simulink library "vmc"  (R2021b)
settings: Solver=VariableStepAuto  StartTime=0.0  StopTime=10.0  RelTol=1e-3
undefined symbols (not defined in the file): AVMC_ACCDeltaTqGradeGn_X_deg, AVMC_ACCDeltaTqIGain4OVRD_X_kph, AVMC_ACCDeltaTqIGain4OVRD_Y_mps2, AVMC_ACCDeltaTqIGain_X_kph, AVMC_ACCDeltaTqIGain_Y_mps2, AVMC_ACCDeltaTqPGain_X_kph, AVMC_ACCDeltaTqPGain_Y_kph, AVMC_ACCGradeofst_X_G, AVMC_ACCGradeofst_Y_pct, AVMC_ACCLoSpdTqLoLim4JP_X_kph, AVMC_ACCLoSpdTqLoLim4JP_Y_deg, AVMC_ACCLoSpdTqLowerLim_X_kph, AVMC_ACCLoSpdTqLowerLim_Y_deg, AVMC_ACCReqAccelGain_X_mps2, AVMC_ACCReqAccelGain_Y_enum, AVMC_ADSPosGFBDeltaTq_X_kph, AVMC_ADSPosGFBDeltaTq_Y_mps2, AVMC_AggressJerkPCT4AT_X_kph, AVMC_AggressJerkPCT_X_kph, AVMC_AggressLimitPCT4AT_X_kph, AVMC_AggressLimitPCT_X_kph, AVMC_DECGradeofst_X_G, AVMC_DECGradeofst_Y_pct, AVMC_DISCDeltaTqIGain_X_kph, AVMC_DISCDeltaTqIGain_Y_mps2, AVMC_DISCDeltaTqPGain_X_kph, AVMC_DISCDeltaTqPGain_Y_kph, AVMC_EPSForceSelect_X_enum, AVMC_EPSForceSelect_Y_enum, AVMC_EPSForceSelectD21_X_enum, AVMC_EPSForceSelectD21_Y_enum, AVMC_ESCRegenOut_X_kph, AVMC_ESCRegenOut_Y_Deg, AVMC_ESCRegenOutEnSpd_X_Deg, AVMC_EstPitchSlopeTs_X_kph, AVMC_GradeCompFlt_X_kph, AVMC_GyroYBandLo_X_Gps, AVMC_HoldResTq_X_kph, AVMC_ISOAccLimit_X_mps, AVMC_ISODecLimit_X_mps, AVMC_ISOJerk_X_mps, AVMC_LatESCRegenOut_X_kph, AVMC_LatESCRegenOut_Y_Deg, AVMC_LongAccDeadZone_X_kph, AVMC_LongAccFiltTsforP2_X_Gps, AVMC_MCPresBaseTq_X_bar, AVMC_MSAPedalOvrd_X_kph, AVMC_MSASpdBand_X_kph, AVMC_MSATqDownEndTq_X_kph, AVMC_MSATqDownTime_X_kph, AVMC_NegZCHoldTq_X_kph, AVMC_OPDDisSlideRate_X_Deg, AVMC_OVRD2ActSR2FCMCMD_X_mps2, AVMC_PedalTqRWhlRatio_X_Nm, AVMC_PedalTqRWhlRatio_Y_gps, AVMC_PedalTqRWhlSlipGain_X_rat, AVMC_PedalTqRWhlSlipGain_Y_kph, AVMC_PedalTqRWhSTRGGain_X_deg, AVMC_PedalTqRWhSTRGGain_Y_kph, AVMC_PosZCHoldTq_X_kph ... (+593)
libraries: hcu_lib x143, simulink x96, tqr x4, $bdroot x1, simulink_extras x1
(part 13 of 17)

== system vmc/VMC/VMC/SPD2ACC/SPD2ACC Active Determination ==
  VVMC_FeatArbitrSta_enum : Inport
  Constant : Constant  Value=TRUE
  Constant1 : Constant  Value=FALSE
  Constant13 : Constant  Value=ENUM_FEATARBITRSTA_DISC
  Constant2 : Constant  Value=ENUM_FEATARBITRSTA_ACCDISC
  Constant3 : Constant  Value=ENUM_FEATARBITRSTA_CC
  Constant4 : Constant  Value=ENUM_FEATARBITRSTA_MSA
  SPD2ACC Active Determination : Stateflow chart  TreatAsAtomicUnit=on
  VVMC_SPD2ACCAct_flg : Outport
  wires:
  Constant4/1 -> SPD2ACC Active Determination/7(ENUM_FEATARBITRSTA_MSA)
  Constant3/1 -> SPD2ACC Active Determination/6(ENUM_FEATARBITRSTA_CC)
  VVMC_FeatArbitrSta_enum/1 -> [VVMC_FeatArbitrSta_enum]
  [VVMC_FeatArbitrSta_enum] -> SPD2ACC Active Determination/1(VVMC_FeatArbitrSta_enum)
  SPD2ACC Active Determination/1(VVMC_SPD2ACCAct_flg) -> [VVMC_SPD2ACCAct_flg]
  [VVMC_SPD2ACCAct_flg] -> VVMC_SPD2ACCAct_flg/1
  Constant/1 -> SPD2ACC Active Determination/2(TURE)
  Constant1/1 -> SPD2ACC Active Determination/3(FALSE)
  Constant13/1 -> SPD2ACC Active Determination/4(ENUM_FEATARBITRSTA_DISC)
  Constant2/1 -> SPD2ACC Active Determination/5(ENUM_FEATARBITRSTA_ACCDISC)

== system vmc/VMC/VMC/SafetyControl/ADB_VehPitchAngleSta ==
  VVMC_CalibratedAccXAftRA_G : Inport
  task_time_s : Inport  Port=2
  VTQD_ExtDoorAllow_flg : Inport  Port=3
  VVMC_VehicleSpeed_kph : Inport  Port=4
  VINP_GRADE_deg : Inport  Port=5
  2-D Lookup Table : Lookup_n-D  BreakpointsForDimension1=AVMC_VehPitchAngleSta_Y_deg  BreakpointsForDimension2=AVMC_VehPitchAngleSta_X_deg  Table=MVMC_VehPitchAngleSta_Z_enum  TableDataTypeStr=uint8  InterpMethod=Flat  InternalRulePriority=Speed  RndMeth=Simplest  InputSameDT=on
      settings: InputPortMap=u0,u1
  AND1 : Logic  AllPortsSameDT=off  OutDataTypeStr=boolean
  Asin : Trigonometry  Operator=asin
  Cast To Single6 : DataTypeConversion  OutDataTypeStr=uint8
  Constant14 : Constant  Value=KVMC_VehStandstillTimer_s
  Constant20 : Constant  Value=KVMC_VehStandstillSpd_kph
  Constant21 : Constant  Value=KVMC_VehPitchAngleMin_deg
  Constant27 : Constant  Value=KVMC_VehPitchAngleMax_deg
  Constant28 : Constant  Value=MINUSONE_FLOAT
  Constant29 : Constant  Value=ONE_FLOAT
  Constant3 : Constant  Value=KVMC_IMUGxFilter4ADB_raw32
  Constant4 : Constant  Value=KVMC_CalEstPitchAngleTs_raw32
  DelayEnable : hcu_lib/Basic_Blocks/DelayEnable
  Detect Increase1 : simulink/Logic and Bit Operations/Detect Increase  vinit=0.0  OutDataTypeStr=boolean
  FirstOrderFilter5 : hcu_lib/Basic_Blocks/FirstOrderFilter
  FirstOrderFilter7 : hcu_lib/Basic_Blocks/FirstOrderFilter
  Gain2 : Gain  Gain=RAD2DEG
  NOT : Logic  Operator=NOT  AllPortsSameDT=off  OutDataTypeStr=boolean
  Relational Operator1 : RelationalOperator  Operator=<  OutDataTypeStr=boolean  RndMeth=Simplest
  Relational Operator2 : RelationalOperator  Operator=<=  OutDataTypeStr=boolean  RndMeth=Simplest
  Relational Operator3 : RelationalOperator  OutDataTypeStr=boolean  RndMeth=Simplest
  SR_Latch4 : hcu_lib/Basic_Blocks/SR_Latch
  Saturation Dynamic3 : simulink/Discontinuities/Saturation Dynamic  OutMin=[]  OutMax=[]  OutDataTypeStr=Inherit: Same as second input  OutDataType=fixdt(1, 16)  OutScaling=2^-10  DoSatur=off
  Switch4 : Switch  Criteria=u2 > Threshold
  Switch5 : Switch  Criteria=u2 > Threshold
  Switch6 : Switch  Criteria=u2 > Threshold
  Unit Delay : UnitDelay  SampleTime=-1  HasFrameUpgradeWarning=on
  VVMC_VehPitchAngleSta_enum : Outport
  wires:
  [VVMC_MemVehPitchAngleEst_deg] -> Switch5/1
  Constant21/1 -> Relational Operator2/2
  Constant14/1 -> DelayEnable/2
  AND1/1 -> NOT/1, SR_Latch4/1
  Unit Delay/1 -> [VVMC_MemVehPitchAngleEst_deg]  "VVMC_MemVehPitchAngleEst_deg"
  Constant4/1 -> FirstOrderFilter7/3
  Constant20/1 -> Relational Operator1/2
  Constant3/1 -> FirstOrderFilter5/3
  FirstOrderFilter7/1 -> Switch4/1  "VVMC_CalEstPitchAngle_deg"
  DelayEnable/1 -> Detect Increase1/1
  Gain2/1 -> FirstOrderFilter7/1
  Asin/1 -> Gain2/1
  Relational Operator3/1 -> Switch6/2
  Switch5/1 -> Switch6/3, Relational Operator3/1
  [VVMC_VehPitchAngleEst_deg] -> 2-D Lookup Table/2
  SR_Latch4/1 -> DelayEnable/1  "VVMC_VehPitchAngleUpdCond_flg"
  [VVMC_VehicleSpeed_kph] -> Relational Operator1/1
  2-D Lookup Table/1 -> Cast To Single6/1
  [VVMC_MemVehPitchAngleEst_deg] -> Switch6/1
  Relational Operator2/1 -> Switch5/2
  Switch4/1 -> Switch5/3, Relational Operator2/1
  Cast To Single6/1 -> [VVMC_VehPitchAngleSta_enum]  "VVMC_VehPitchAngleSta_enum"
  Relational Operator1/1 -> AND1/2
  Switch6/1 -> Unit Delay/1, [VVMC_VehPitchAngleEst_deg]  "VVMC_VehPitchAngleEst_deg"
  [task_time_s] -> FirstOrderFilter7/2
  Detect Increase1/1 -> Switch4/2  "VVMC_VehPitchAngleUpd_flg"
  [VTQD_ExtDoorAllow_flg] -> AND1/1
  [task_time_s] -> DelayEnable/3
  [VVMC_MemVehPitchAngleEst_deg] -> Switch4/3
  [VVMC_CalibratedAccXAftRA_G] -> FirstOrderFilter5/1
  [VINP_GRADE_deg] -> 2-D Lookup Table/1
  [task_time_s] -> FirstOrderFilter5/2
  NOT/1 -> SR_Latch4/2
  Constant27/1 -> Relational Operator3/2
  [VVMC_VehPitchAngleSta_enum] -> VVMC_VehPitchAngleSta_enum/1
  VVMC_CalibratedAccXAftRA_G/1 -> [VVMC_CalibratedAccXAftRA_G]
  task_time_s/1 -> [task_time_s]
  VTQD_ExtDoorAllow_flg/1 -> [VTQD_ExtDoorAllow_flg]
  VVMC_VehicleSpeed_kph/1 -> [VVMC_VehicleSpeed_kph]
  VINP_GRADE_deg/1 -> [VINP_GRADE_deg]
  Constant29/1 -> Saturation Dynamic3/1
  Constant28/1 -> Saturation Dynamic3/3
  FirstOrderFilter5/1 -> Saturation Dynamic3/2
  Saturation Dynamic3/1 -> Asin/1

== system vmc/VMC/VMC/SafetyControl/LatAccRollingAverage ==
  VINP_LatAccel_Gps : Inport
  VINP_LatAccelV_flg : Inport  Port=2
  VDDM_ESC5Err_flg : Inport  Port=3
  Cast To Single4 : DataTypeConversion  OutDataTypeStr=uint8
  Constant15 : Constant  Value=ZERO_FLOAT
  Constant3 : Constant  Value=ONE_INT
  Constant4 : Constant  Value=ZERO_FLOAT
  Constant5 : Constant  Value=KVMC_LatAccRollAveLevel_enum
  Constant6 : Constant  Value=ONE_INT
  Min2 : MinMax  Function=max  Inputs=2
  OR2 : Logic  Operator=OR  AllPortsSameDT=off  OutDataTypeStr=boolean
  RollingAverage : Stateflow chart  TreatAsAtomicUnit=on
  Switch2 : Switch  Criteria=u2 > Threshold
  VVMC_LatAccRollAveRaw_Gps : Outport
  wires:
  [VDDM_ESC5Err_flg] -> OR2/2
  OR2/1 -> Switch2/2
  VDDM_ESC5Err_flg/1 -> [VDDM_ESC5Err_flg]
  [VINP_LatAccel_Gps] -> Switch2/3
  Constant15/1 -> Switch2/1
  [VINP_LatAccelV_flg] -> OR2/1
  VINP_LatAccelV_flg/1 -> [VINP_LatAccelV_flg]
  Cast To Single4/1 -> Min2/1
  Constant5/1 -> Cast To Single4/1
  Constant6/1 -> Min2/2
  Switch2/1 -> RollingAverage/4(VINP_LatAccel_Gps)
  Constant4/1 -> RollingAverage/2(ZERO_FLOAT)
  Constant3/1 -> RollingAverage/3(ONE_INT)
  Min2/1 -> RollingAverage/1(KVMC_LatAccRollAveLevel_enum)
  [VVMC_LatAccRollAveRaw_Gps] -> VVMC_LatAccRollAveRaw_Gps/1
  VINP_LatAccel_Gps/1 -> [VINP_LatAccel_Gps]
  RollingAverage/1(VVMC_LatAccRollAveRaw_Gps) -> [VVMC_LatAccRollAveRaw_Gps]  "VVMC_LatAccRollAveRaw_Gps"

== system vmc/VMC/VMC/SafetyControl/LongAccel_EstSlope_FrontRearSlipSpd ==
  VVMC_VehSpdRollAve_kph : Inport
  VVMC_CalibratedAccX_G : Inport  Port=2
  VVMC_IMUEnaCmd_flg : Inport  Port=3
  VINP_LongAccel_Gps : Inport  Port=4
  VINP_GRADE_deg : Inport  Port=5
  VVMC_LFWhlSpeedRollAve_kph : Inport  Port=6
  VVMC_RFWhlSpeedRollAve_kph : Inport  Port=7
  VVMC_LRWhlSpeedRollAve_kph : Inport  Port=8
  VVMC_RRWhlSpeedRollAve_kph : Inport  Port=9
  VINP_LFRawWhlSpeedV_flg : Inport  Port=10
  VINP_RFRawWhlSpeedV_flg : Inport  Port=11
  VINP_LRRawWhlSpeedV_flg : Inport  Port=12
  VINP_RRRawWhlSpeedV_flg : Inport  Port=13
  VVMC_VehicleSpeed_kph : Inport  Port=14
  task_time_s : Inport  Port=15
  AND : Logic  AllPortsSameDT=off  OutDataTypeStr=boolean
  Add1 : Sum
  Add10 : Sum  Inputs=+-
  Add9 : Sum
  Constant : Constant  Tag=struct('comment',struct('text','','placement',1),'output',struct('width',1,'name','$S_$B','unit','','type','Int16','offset',0,'max',NaN,'min',NaN,'freeze',1,'lsb',1,'arb',0,'class','default','address','','description','','value','0','tolerance',1,'show',0),'date',731450.689904282)  Value=ZERO_FLOAT  OutDataTypeStr=single
  Constant1 : Constant  Value=KVMC_LongAccelDiffTime_s
  Constant10 : Constant  Value=KVMC_LongAccelDiffTime_s
  Constant11 : Constant  Value=GRAVITY_G
  Constant12 : Constant  Value=KPH2MPS
  Constant13 : Constant  Tag=struct('comment',struct('text','','placement',1),'output',struct('width',1,'name','$S_$B','unit','','type','Int16','offset',0,'max',NaN,'min',NaN,'freeze',1,'lsb',1,'arb',0,'class','default','address','','description','','value','2','tolerance',1,'show',0),'date',731450.690075)  Value=TRUE
  Constant18 : Constant  Value=TWO_FLOAT
  Constant19 : Constant  Value=TWO_FLOAT
  Constant2 : Constant  Value=ZERO_FLOAT
  Constant24 : Constant  Value=GRAVITY_G
  Constant25 : Constant  Value=KPH2MPS
  Constant28 : Constant  Value=KVMC_EstSlopeGxSource_flg
  Constant3 : Constant  Tag=struct('comment',struct('text','','placement',1),'output',struct('width',1,'name','$S_$B','unit','','type','Int16','offset',0,'max',NaN,'min',NaN,'freeze',1,'lsb',1,'arb',0,'class','default','address','','description','','value','0','tolerance',1,'show',0),'date',731450.689904282)  Value=ZERO_FLOAT  OutDataTypeStr=single
  Constant4 : Constant  Value=KVMC_LongAccelDiffTime_s
  Constant5 : Constant  Tag=struct('comment',struct('text','','placement',1),'output',struct('width',1,'name','$S_$B','unit','','type','Int16','offset',0,'max',NaN,'min',NaN,'freeze',1,'lsb',1,'arb',0,'class','default','address','','description','','value','2','tolerance',1,'show',0),'date',731450.690075)  Value=TRUE
  Constant6 : Constant  Value=GRAVITY_G
  Constant7 : Constant  Value=KPH2MPS
  Constant8 : Constant  Tag=struct('comment',struct('text','','placement',1),'output',struct('width',1,'name','$S_$B','unit','','type','Int16','offset',0,'max',NaN,'min',NaN,'freeze',1,'lsb',1,'arb',0,'class','default','address','','description','','value','2','tolerance',1,'show',0),'date',731450.690075)  Value=TRUE
  Constant9 : Constant  Tag=struct('comment',struct('text','','placement',1),'output',struct('width',1,'name','$S_$B','unit','','type','Int16','offset',0,'max',NaN,'min',NaN,'freeze',1,'lsb',1,'arb',0,'class','default','address','','description','','value','0','tolerance',1,'show',0),'date',731450.689904282)  Value=ZERO_FLOAT  OutDataTypeStr=single
  Divide1 : Product  Inputs=**
  Divide2 : Product  Inputs=**
  Divide{3..6,8} (5 alike) : Product  Inputs=*/
  Divide7 : Product  Inputs=**
  Estimate Slope : Subsystem
  Max : MinMax  Function=max  Inputs=2
  Max1 : MinMax  Function=max  Inputs=2
  Max2 : MinMax  Function=max  Inputs=2
  OR1 : Logic  Operator=OR  AllPortsSameDT=off  OutDataTypeStr=boolean
  OR2 : Logic  Operator=OR  AllPortsSameDT=off  OutDataTypeStr=boolean
  OR3 : Logic  AllPortsSameDT=off  OutDataTypeStr=boolean
  OR4 : Logic  AllPortsSameDT=off  OutDataTypeStr=boolean
  OR5 : Logic  Operator=OR  AllPortsSameDT=off  OutDataTypeStr=boolean
  Product : Product  Tag=struct('comment',struct('text','','placement',1),'logdata',struct('maxnumvals',inf,'plotchannels',[],'stepsize',0,'downsampling',1,'loggingmode',3,'channels',1),'output',struct('width',1,'name','$S_$B','unit','','type','Int32Bin15','offset',0,'max',65535,'min',-65536,'freeze',1,'lsb',2^-15,'arb',0,'class','default','address','','description','','autoscalingmode',1,'lowerheadroom',1,'upperheadroom',1,'headroomunit','bit','checkmin',0,'checkmax',0,'show',0),'inputs','*/','exceptionhandling',1,'date',731458.438505301)  Inputs=*/  InputSameDT=on  RndMeth=Zero  SaturateOnIntegerOverflow=on  OutDataTypeStr=Inherit: Same as first input
  Product1 : Product  Tag=struct('comment',struct('text','','placement',1),'logdata',struct('maxnumvals',inf,'plotchannels',[],'stepsize',0,'downsampling',1,'loggingmode',3,'channels',1),'output',struct('width',1,'name','$S_$B','unit','','type','Int32Bin15','offset',0,'max',65535,'min',-65536,'freeze',1,'lsb',2^-15,'arb',0,'class','default','address','','description','','autoscalingmode',1,'lowerheadroom',1,'upperheadroom',1,'headroomunit','bit','checkmin',0,'checkmax',0,'show',0),'inputs','*/','exceptionhandling',1,'date',731458.438505301)  Inputs=*/  InputSameDT=on  RndMeth=Zero  SaturateOnIntegerOverflow=on  OutDataTypeStr=Inherit: Same as first input
  Product2 : Product  Tag=struct('comment',struct('text','','placement',1),'logdata',struct('maxnumvals',inf,'plotchannels',[],'stepsize',0,'downsampling',1,'loggingmode',3,'channels',1),'output',struct('width',1,'name','$S_$B','unit','','type','Int32Bin15','offset',0,'max',65535,'min',-65536,'freeze',1,'lsb',2^-15,'arb',0,'class','default','address','','description','','autoscalingmode',1,'lowerheadroom',1,'upperheadroom',1,'headroomunit','bit','checkmin',0,'checkmax',0,'show',0),'inputs','*/','exceptionhandling',1,'date',731458.438505301)  Inputs=*/  InputSameDT=on  RndMeth=Zero  SaturateOnIntegerOverflow=on  OutDataTypeStr=Inherit: Same as first input
  Sum : Sum  Tag=struct('comment',struct('text','','placement',1),'logdata',struct('maxnumvals',inf,'plotchannels',[],'stepsize',0,'downsampling',1,'loggingmode',3,'channels',1),'output',struct('width',1,'name','$S_$B','unit','','type','Int32Bin15','offset',0,'max',65535,'min',-65536,'freeze',1,'lsb',2^-15,'arb',0,'class','default','address','','description','','autoscalingmode',1,'lowerheadroom',1,'upperheadroom',1,'headroomunit','bit','checkmin',0,'checkmax',0,'show',0),'inputs','+-','date',731450.688943275)  Inputs=+-  InputSameDT=on  SaturateOnIntegerOverflow=on  OutDataTypeStr=Inherit: Same as first input
  Sum1 : Sum  Tag=struct('comment',struct('text','','placement',1),'logdata',struct('maxnumvals',inf,'plotchannels',[],'stepsize',0,'downsampling',1,'loggingmode',3,'channels',1),'output',struct('width',1,'name','$S_$B','unit','','type','Int32Bin15','offset',0,'max',65535,'min',-65536,'freeze',1,'lsb',2^-15,'arb',0,'class','default','address','','description','','autoscalingmode',1,'lowerheadroom',1,'upperheadroom',1,'headroomunit','bit','checkmin',0,'checkmax',0,'show',0),'inputs','+-','date',731450.688943275)  Inputs=+-  InputSameDT=on  SaturateOnIntegerOverflow=on  OutDataTypeStr=Inherit: Same as first input
  Sum2 : Sum  Tag=struct('comment',struct('text','','placement',1),'logdata',struct('maxnumvals',inf,'plotchannels',[],'stepsize',0,'downsampling',1,'loggingmode',3,'channels',1),'output',struct('width',1,'name','$S_$B','unit','','type','Int32Bin15','offset',0,'max',65535,'min',-65536,'freeze',1,'lsb',2^-15,'arb',0,'class','default','address','','description','','autoscalingmode',1,'lowerheadroom',1,'upperheadroom',1,'headroomunit','bit','checkmin',0,'checkmax',0,'show',0),'inputs','+-','date',731450.688943275)  Inputs=+-  InputSameDT=on  SaturateOnIntegerOverflow=on  OutDataTypeStr=Inherit: Same as first input
  Switch{,1..3} (4 alike) : Switch  Criteria=u2 > Threshold
  Switch4 : Switch  Tag=struct('comment',struct('text','','placement',1),'logdata',struct('maxnumvals',inf,'plotchannels',[],'stepsize',0,'downsampling',1,'loggingmode',3,'channels',1),'output',struct('width',1,'name','$S_$B','unit','','type','Int32Bin15','offset',0,'max',65535,'min',-65536,'freeze',1,'lsb',2^-15,'arb',0,'class','default','address','','description','','autoscalingmode',1,'lowerheadroom',1,'upperheadroom',1,'headroomunit','bit','checkmin',0,'checkmax',0,'show',0),'threshold',struct('width',1,'name','$S_$B_threshold','unit','','type','Int16','offset',0,'max',NaN,'min',NaN,'freeze',1,'lsb',1,'arb',0,'class','default','address','','description','','value','1','scalar',0),'date',731458.438569977)  Criteria=u2 > Threshold  SaturateOnIntegerOverflow=on  InputSameDT=on
  Switch5 : Switch  Tag=struct('comment',struct('text','','placement',1),'logdata',struct('maxnumvals',inf,'plotchannels',[],'stepsize',0,'downsampling',1,'loggingmode',3,'channels',1),'output',struct('width',1,'name','$S_$B','unit','','type','Int32Bin15','offset',0,'max',65535,'min',-65536,'freeze',1,'lsb',2^-15,'arb',0,'class','default','address','','description','','autoscalingmode',1,'lowerheadroom',1,'upperheadroom',1,'headroomunit','bit','checkmin',0,'checkmax',0,'show',0),'threshold',struct('width',1,'name','$S_$B_threshold','unit','','type','Int16','offset',0,'max',NaN,'min',NaN,'freeze',1,'lsb',1,'arb',0,'class','default','address','','description','','value','1','scalar',0),'date',731458.438569977)  Criteria=u2 > Threshold  SaturateOnIntegerOverflow=on  InputSameDT=on
  Switch6 : Switch  Tag=struct('comment',struct('text','','placement',1),'logdata',struct('maxnumvals',inf,'plotchannels',[],'stepsize',0,'downsampling',1,'loggingmode',3,'channels',1),'output',struct('width',1,'name','$S_$B','unit','','type','Int32Bin15','offset',0,'max',65535,'min',-65536,'freeze',1,'lsb',2^-15,'arb',0,'class','default','address','','description','','autoscalingmode',1,'lowerheadroom',1,'upperheadroom',1,'headroomunit','bit','checkmin',0,'checkmax',0,'show',0),'threshold',struct('width',1,'name','$S_$B_threshold','unit','','type','Int16','offset',0,'max',NaN,'min',NaN,'freeze',1,'lsb',1,'arb',0,'class','default','address','','description','','value','1','scalar',0),'date',731458.438569977)  Criteria=u2 > Threshold  SaturateOnIntegerOverflow=on  InputSameDT=on
  UnitDelay1 : UnitDelay  Tag=struct('comment',struct('text','','placement',1),'logdata',struct('maxnumvals',inf,'plotchannels',[],'stepsize',0,'downsampling',1,'loggingmode',3,'channels',1),'output',struct('width',1,'name','$S_$B','unit','','type','Int32Bin15','offset',0,'max',65535,'min',-65536,'freeze',1,'lsb',2^-15,'arb',0,'class','default','address','','description','','autoscalingmode',1,'lowerheadroom',1,'upperheadroom',1,'headroomunit','bit','checkmin',0,'checkmax',0,'show',0,'initial','0'),'state',0,'dt','-1','date',731450.687911019)  SampleTime=-1  HasFrameUpgradeWarning=on
  UnitDelay2 : UnitDelay  Tag=struct('comment',struct('text','','placement',1),'logdata',struct('maxnumvals',inf,'plotchannels',[],'stepsize',0,'downsampling',1,'loggingmode',3,'channels',1),'output',struct('width',1,'name','$S_$B','unit','','type','UInt8','offset',0,'max',255,'min',0,'freeze',1,'lsb',1,'arb',0,'class','default','address','','description','','autoscalingmode',1,'lowerheadroom',1,'upperheadroom',1,'headroomunit','bit','checkmin',0,'checkmax',0,'show',0,'initial','0'),'state',0,'dt','-1','date',731450.690382801)  InitialCondition=FALSE  SampleTime=-1  StateName=first_pass  HasFrameUpgradeWarning=on
  UnitDelay3 : UnitDelay  Tag=struct('comment',struct('text','','placement',1),'logdata',struct('maxnumvals',inf,'plotchannels',[],'stepsize',0,'downsampling',1,'loggingmode',3,'channels',1),'output',struct('width',1,'name','$S_$B','unit','','type','Int32Bin15','offset',0,'max',65535,'min',-65536,'freeze',1,'lsb',2^-15,'arb',0,'class','default','address','','description','','autoscalingmode',1,'lowerheadroom',1,'upperheadroom',1,'headroomunit','bit','checkmin',0,'checkmax',0,'show',0,'initial','0'),'state',0,'dt','-1','date',731450.687911019)  SampleTime=-1  HasFrameUpgradeWarning=on
  UnitDelay4 : UnitDelay  Tag=struct('comment',struct('text','','placement',1),'logdata',struct('maxnumvals',inf,'plotchannels',[],'stepsize',0,'downsampling',1,'loggingmode',3,'channels',1),'output',struct('width',1,'name','$S_$B','unit','','type','UInt8','offset',0,'max',255,'min',0,'freeze',1,'lsb',1,'arb',0,'class','default','address','','description','','autoscalingmode',1,'lowerheadroom',1,'upperheadroom',1,'headroomunit','bit','checkmin',0,'checkmax',0,'show',0,'initial','0'),'state',0,'dt','-1','date',731450.690382801)  InitialCondition=FALSE  SampleTime=-1  StateName=first_pass  HasFrameUpgradeWarning=on
  UnitDelay5 : UnitDelay  Tag=struct('comment',struct('text','','placement',1),'logdata',struct('maxnumvals',inf,'plotchannels',[],'stepsize',0,'downsampling',1,'loggingmode',3,'channels',1),'output',struct('width',1,'name','$S_$B','unit','','type','Int32Bin15','offset',0,'max',65535,'min',-65536,'freeze',1,'lsb',2^-15,'arb',0,'class','default','address','','description','','autoscalingmode',1,'lowerheadroom',1,'upperheadroom',1,'headroomunit','bit','checkmin',0,'checkmax',0,'show',0,'initial','0'),'state',0,'dt','-1','date',731450.687911019)  SampleTime=-1  HasFrameUpgradeWarning=on
  UnitDelay6 : UnitDelay  Tag=struct('comment',struct('text','','placement',1),'logdata',struct('maxnumvals',inf,'plotchannels',[],'stepsize',0,'downsampling',1,'loggingmode',3,'channels',1),'output',struct('width',1,'name','$S_$B','unit','','type','UInt8','offset',0,'max',255,'min',0,'freeze',1,'lsb',1,'arb',0,'class','default','address','','description','','autoscalingmode',1,'lowerheadroom',1,'upperheadroom',1,'headroomunit','bit','checkmin',0,'checkmax',0,'show',0,'initial','0'),'state',0,'dt','-1','date',731450.690382801)  InitialCondition=FALSE  SampleTime=-1  StateName=first_pass  HasFrameUpgradeWarning=on
  VVMC_LongAccelCalcuByVehSpdRaw_gps : Outport
  VVMC_EstSlopeCal_Deg : Outport  Port=2
  VVMC_FrRrSlipSpd_kph : Outport  Port=3
  VVMC_LongAccelCalcuFrWhlRaw_gps : Outport  Port=4
  VVMC_LongAccelCalcuRrWhlRaw_gps : Outport  Port=5
  VVMC_FrWhlSpdInvalid_flg : Outport  Port=6
  VVMC_RrWhlSpdInvalid_flg : Outport  Port=7
  wires:
  [VVMC_IMUEnaCmd_flg] -> AND/1
  [VVMC_RrWhlSpdInvalid_flg] -> Switch2/2
  [VINP_RFRawWhlSpeedV_flg] -> OR4/2
  [VINP_LRRawWhlSpeedV_flg] -> OR2/1
  OR4/1 -> OR5/1
  OR5/1 -> Switch3/2
  [VVMC_CalibratedAccX_G] -> Switch/1
  Add10/1 -> Switch3/3
  [VINP_RRRawWhlSpeedV_flg] -> OR2/2
  AND/1 -> Switch/2
  [VINP_GRADE_deg] -> Estimate Slope/3(VINP_GRADE_deg)
  [VINP_LFRawWhlSpeedV_flg] -> OR1/1
  [VINP_LFRawWhlSpeedV_flg] -> OR4/1
  [VVMC_VehSpdRollAve_kph] -> Divide2/1
  Constant2/1 -> Switch3/1
  OR3/1 -> OR5/2
  Switch3/1 -> [VVMC_FrRrSlipSpd_kph]  "VVMC_FrRrSlipSpd_kph"
  Constant28/1 -> AND/2
  Switch/1 -> Estimate Slope/1(VINP_LongAccel_Gps)
  Add9/1 -> Divide6/1, Switch2/1
  [VVMC_VehicleSpeed_kph] -> Estimate Slope/2(VVMC_VehicleSpeed_kph)
  Switch1/1 -> Add10/1
  Divide5/1 -> Switch1/3, [VVMC_FrWhlSpdRollAve_kph]  "VVMC_FrWhlSpdRollAve_kph"
  Switch2/1 -> Add10/2
  Product/1 -> Divide4/1
  [VINP_LongAccel_Gps] -> Switch/3
  Constant24/1 -> Divide4/2
  [VVMC_LRWhlSpeedRollAve_kph] -> Add9/1
  Constant25/1 -> Divide2/2
  Divide6/1 -> [VVMC_RrWhlSpdRollAve_kph], Switch2/3  "VVMC_RrWhlSpdRollAve_kph"
  Constant19/1 -> Divide6/2
  Divide4/1 -> [VVMC_LongAccelCalcuByVehSpdRaw_gps]  "VVMC_LongAccelCalcuByVehSpdRaw_gps"
  Estimate Slope/1(VVMC_EstSlopeCal_Deg) -> [VVMC_EstSlopeCal_Deg]
  [VINP_RFRawWhlSpeedV_flg] -> OR1/2
  Constant1/1 -> Max/1
  [VVMC_RRWhlSpeedRollAve_kph] -> Add9/2
  Add1/1 -> Divide5/1, Switch1/1
  [VVMC_FrWhlSpdInvalid_flg] -> Switch1/2
  [VINP_RRRawWhlSpeedV_flg] -> OR3/2
  Constant18/1 -> Divide5/2
  [VVMC_RFWhlSpeedRollAve_kph] -> Add1/2
  [VVMC_LFWhlSpeedRollAve_kph] -> Add1/1
  [VINP_LRRawWhlSpeedV_flg] -> OR3/1
  VVMC_VehSpdRollAve_kph/1 -> [VVMC_VehSpdRollAve_kph]
  VVMC_CalibratedAccX_G/1 -> [VVMC_CalibratedAccX_G]
  VVMC_IMUEnaCmd_flg/1 -> [VVMC_IMUEnaCmd_flg]
  VINP_LongAccel_Gps/1 -> [VINP_LongAccel_Gps]
  VINP_GRADE_deg/1 -> [VINP_GRADE_deg]
  VVMC_LFWhlSpeedRollAve_kph/1 -> [VVMC_LFWhlSpeedRollAve_kph]
  VVMC_RFWhlSpeedRollAve_kph/1 -> [VVMC_RFWhlSpeedRollAve_kph]
  VVMC_LRWhlSpeedRollAve_kph/1 -> [VVMC_LRWhlSpeedRollAve_kph]
  VVMC_RRWhlSpeedRollAve_kph/1 -> [VVMC_RRWhlSpeedRollAve_kph]
  VINP_LFRawWhlSpeedV_flg/1 -> [VINP_LFRawWhlSpeedV_flg]
  VINP_RFRawWhlSpeedV_flg/1 -> [VINP_RFRawWhlSpeedV_flg]
  VINP_LRRawWhlSpeedV_flg/1 -> [VINP_LRRawWhlSpeedV_flg]
  VINP_RRRawWhlSpeedV_flg/1 -> [VINP_RRRawWhlSpeedV_flg]
  [VVMC_LongAccelCalcuByVehSpdRaw_gps] -> VVMC_LongAccelCalcuByVehSpdRaw_gps/1
  [VVMC_EstSlopeCal_Deg] -> VVMC_EstSlopeCal_Deg/1
  [VVMC_FrRrSlipSpd_kph] -> VVMC_FrRrSlipSpd_kph/1
  VVMC_VehicleSpeed_kph/1 -> [VVMC_VehicleSpeed_kph]
  [task_time_s] -> Estimate Slope/4(task_time_s)
  task_time_s/1 -> [task_time_s]
  UnitDelay1/1 -> Sum/2
  Constant5/1 -> UnitDelay2/1
  Switch4/1 -> Product/1
  UnitDelay2/1 -> Switch4/2
  Constant/1 -> Switch4/3
  Sum/1 -> Switch4/1
  Divide2/1 -> UnitDelay1/1, Sum/1
  Max/1 -> Product/2
  [task_time_s] -> Max/2
  [task_time_s] -> Max1/2
  Max1/1 -> Product1/2
  Divide1/1 -> Sum1/1, UnitDelay3/1
  Sum1/1 -> Switch5/1
  Constant3/1 -> Switch5/3
  UnitDelay4/1 -> Switch5/2
  Switch5/1 -> Product1/1
  Constant8/1 -> UnitDelay4/1
  UnitDelay3/1 -> Sum1/2
  Constant4/1 -> Max1/1
  Divide3/1 -> [VVMC_LongAccelCalcuFrWhlRaw_gps]  "VVMC_LongAccelCalcuFrWhlRaw_gps"
  Constant7/1 -> Divide1/2
  Constant6/1 -> Divide3/2
  Product1/1 -> Divide3/1
  [VVMC_FrWhlSpdRollAve_kph] -> Divide1/1
  [VVMC_RrWhlSpdRollAve_kph] -> Divide7/1
  Product2/1 -> Divide8/1
  Constant11/1 -> Divide8/2
  Constant12/1 -> Divide7/2
  Divide8/1 -> [VVMC_LongAccelCalcuRrWhlRaw_gps]  "VVMC_LongAccelCalcuRrWhlRaw_gps"
  Constant10/1 -> Max2/1
  UnitDelay5/1 -> Sum2/2
  Constant13/1 -> UnitDelay6/1
  Switch6/1 -> Product2/1
  UnitDelay6/1 -> Switch6/2
  Constant9/1 -> Switch6/3
  Sum2/1 -> Switch6/1
  Divide7/1 -> UnitDelay5/1, Sum2/1
  Max2/1 -> Product2/2
  [task_time_s] -> Max2/2
  [VVMC_LongAccelCalcuFrWhlRaw_gps] -> VVMC_LongAccelCalcuFrWhlRaw_gps/1
  [VVMC_LongAccelCalcuRrWhlRaw_gps] -> VVMC_LongAccelCalcuRrWhlRaw_gps/1
  OR1/1 -> [VVMC_FrWhlSpdInvalid_flg]  "VVMC_FrWhlSpdInvalid_flg"
  OR2/1 -> [VVMC_RrWhlSpdInvalid_flg]  "VVMC_RrWhlSpdInvalid_flg"
  [VVMC_FrWhlSpdInvalid_flg] -> VVMC_FrWhlSpdInvalid_flg/1
  [VVMC_RrWhlSpdInvalid_flg] -> VVMC_RrWhlSpdInvalid_flg/1

== system vmc/VMC/VMC/SafetyControl/Rolling Average Engage ==
  task_time_s : Inport
  Add2 : Sum
  Constant5 : Constant  Value=KVMC_RollAveEnTime_s
  Min1 : MinMax  Inputs=2
  Relational Operator : RelationalOperator  OutDataTypeStr=boolean  RndMeth=Simplest
  initial: 0 : UnitDelay  SampleTime=-1  HasFrameUpgradeWarning=on
  VVMC_RollAveEn_flg : Outport
  wires:
  Min1/1 -> Relational Operator/1, initial: 0/1
  Constant5/1 -> Relational Operator/2, Min1/2
  Add2/1 -> Min1/1
  Relational Operator/1 -> VVMC_RollAveEn_flg/1  "VVMC_RollAveEn_flg"
  task_time_s/1 -> Add2/2
  initial: 0/1 -> Add2/1

== system vmc/VMC/VMC/SafetyControl/SafetyControlJudgement ==
  VVMC_VehicleSpeed_kph : Inport
  VVMC_LFWhlSpeedRollAve_kph : Inport  Port=2
  VVMC_RFWhlSpeedRollAve_kph : Inport  Port=3
  VVMC_LRWhlSpeedRollAve_kph : Inport  Port=4
  VVMC_RRWhlSpeedRollAve_kph : Inport  Port=5
  VINP_LFRawWhlSpeedV_flg : Inport  Port=6
  VINP_RFRawWhlSpeedV_flg : Inport  Port=7
  VINP_LRRawWhlSpeedV_flg : Inport  Port=8
  VINP_RRRawWhlSpeedV_flg : Inport  Port=9
  VVMC_LatAccRollAve_Gps : Inport  Port=10
  VINP_LatAccelV_flg : Inport  Port=11
  VVMC_FeatArbitrFinal_enum : Inport  Port=12
  task_time_s : Inport  Port=13
  Cast To Single{,1..3} (4 alike) : DataTypeConversion  OutDataTypeStr=boolean
  Constant20 : Constant  Value=KVMC_SafetyCtrlAllowTime_s
  Constant21 : Constant  Value=TRUE
  Constant22 : Constant  Value=FALSE
  FrontRearSlipRatio : Subsystem
  LateralAccelerationControl : Subsystem
  NOT : Logic  Operator=NOT  AllPortsSameDT=off  OutDataTypeStr=boolean
  RearWheelSlipRatio : Subsystem
  Relational Operator16 : RelationalOperator  OutDataTypeStr=boolean  RndMeth=Simplest
  SafetyControlJudgement : Subsystem
  SingleWheelSlipRatio : Subsystem
  Timer : hcu_lib/Basic_Blocks/Timer
  u2 > 0 (1) : Switch  Criteria=u2 > Threshold
  VVMC_SafetyCtrl_flg : Outport
  VVMC_FrontRearSlipRatioCtrl_flg : Outport  Port=2
  VVMC_RearWhlSlipRatioCtrl_flg : Outport  Port=3
  VVMC_SingleWhlSlipRatioCtrl_flg : Outport  Port=4
  VVMC_LatAccCtrl_flg : Outport  Port=5
  wires:
  VVMC_VehicleSpeed_kph/1 -> [VVMC_VehicleSpeed_kph]
  VVMC_RRWhlSpeedRollAve_kph/1 -> [VVMC_RRWhlSpeedRollAve_kph]
  VVMC_LRWhlSpeedRollAve_kph/1 -> [VVMC_LRWhlSpeedRollAve_kph]
  VVMC_RFWhlSpeedRollAve_kph/1 -> [VVMC_RFWhlSpeedRollAve_kph]
  VVMC_LFWhlSpeedRollAve_kph/1 -> [VVMC_LFWhlSpeedRollAve_kph]
  VINP_LFRawWhlSpeedV_flg/1 -> [VINP_LFRawWhlSpeedV_flg]
  VINP_RFRawWhlSpeedV_flg/1 -> [VINP_RFRawWhlSpeedV_flg]
  VINP_LRRawWhlSpeedV_flg/1 -> [VINP_LRRawWhlSpeedV_flg]
  VINP_RRRawWhlSpeedV_flg/1 -> [VINP_RRRawWhlSpeedV_flg]
  [VVMC_LFWhlSpeedRollAve_kph] -> FrontRearSlipRatio/1(VVMC_LFWhlSpeedRollAve_kph)
  [VVMC_RFWhlSpeedRollAve_kph] -> FrontRearSlipRatio/2(VVMC_RFWhlSpeedRollAve_kph)
  [VVMC_LRWhlSpeedRollAve_kph] -> FrontRearSlipRatio/3(VVMC_LRWhlSpeedRollAve_kph)
  [VVMC_RRWhlSpeedRollAve_kph] -> FrontRearSlipRatio/4(VVMC_RRWhlSpeedRollAve_kph)
  [VINP_LFRawWhlSpeedV_flg] -> FrontRearSlipRatio/5(VINP_LFRawWhlSpeedV_flg)
  [VINP_RFRawWhlSpeedV_flg] -> FrontRearSlipRatio/6(VINP_RFRawWhlSpeedV_flg)
  [VINP_LRRawWhlSpeedV_flg] -> FrontRearSlipRatio/7(VINP_LRRawWhlSpeedV_flg)
  [VINP_RRRawWhlSpeedV_flg] -> FrontRearSlipRatio/8(VINP_RRRawWhlSpeedV_flg)
  FrontRearSlipRatio/1("VVMC_FrontRearSlipRatioCtrl_flg ") -> Cast To Single/1
  RearWheelSlipRatio/1("VVMC_RearWhlSlipRatioCtrl_flg ") -> Cast To Single1/1
  [VINP_RRRawWhlSpeedV_flg] -> RearWheelSlipRatio/4(VINP_RRRawWhlSpeedV_flg)
  [VINP_LRRawWhlSpeedV_flg] -> RearWheelSlipRatio/3(VINP_LRRawWhlSpeedV_flg)
  [VVMC_RRWhlSpeedRollAve_kph] -> RearWheelSlipRatio/2(VVMC_RRWhlSpeedRollAve_kph)
  [VVMC_LRWhlSpeedRollAve_kph] -> RearWheelSlipRatio/1(VVMC_LRWhlSpeedRollAve_kph)
  SingleWheelSlipRatio/1(VVMC_SingleWhlSlipRatioCtrl_flg) -> Cast To Single2/1
  [VINP_RRRawWhlSpeedV_flg] -> SingleWheelSlipRatio/9(VINP_RRRawWhlSpeedV_flg)
  [VINP_LRRawWhlSpeedV_flg] -> SingleWheelSlipRatio/8(VINP_LRRawWhlSpeedV_flg)
  [VINP_RFRawWhlSpeedV_flg] -> SingleWheelSlipRatio/7(VINP_RFRawWhlSpeedV_flg)
  [VINP_LFRawWhlSpeedV_flg] -> SingleWheelSlipRatio/6(VINP_LFRawWhlSpeedV_flg)
  [VVMC_RRWhlSpeedRollAve_kph] -> SingleWheelSlipRatio/5(VVMC_RRWhlSpeedRollAve_kph)
  [VVMC_LRWhlSpeedRollAve_kph] -> SingleWheelSlipRatio/4(VVMC_LRWhlSpeedRollAve_kph)
  [VVMC_RFWhlSpeedRollAve_kph] -> SingleWheelSlipRatio/3(VVMC_RFWhlSpeedRollAve_kph)
  [VVMC_LFWhlSpeedRollAve_kph] -> SingleWheelSlipRatio/2(VVMC_LFWhlSpeedRollAve_kph)
  [VVMC_VehicleSpeed_kph] -> SingleWheelSlipRatio/1(VVMC_VehicleSpeed_kph)
  [VVMC_FrontRearSlipRatioCtrl_flg] -> SafetyControlJudgement/1(VVMC_FrontRearSlipRatioCtrl_flg)
  [VVMC_RearWhlSlipRatioCtrl_flg] -> SafetyControlJudgement/2(VVMC_RearWhlSlipRatioCtrl_flg)
  [VVMC_SingleWhlSlipRatioCtrl_flg] -> SafetyControlJudgement/3(VVMC_SingleWhlSlipRatioCtrl_flg)
  [VVMC_SafetyCtrl_flg] -> VVMC_SafetyCtrl_flg/1
  Cast To Single/1 -> [VVMC_FrontRearSlipRatioCtrl_flg]  "VVMC_FrontRearSlipRatioCtrl_flg"
  Cast To Single1/1 -> [VVMC_RearWhlSlipRatioCtrl_flg]  "VVMC_RearWhlSlipRatioCtrl_flg"
  Cast To Single2/1 -> [VVMC_SingleWhlSlipRatioCtrl_flg]  "VVMC_SingleWhlSlipRatioCtrl_flg"
  VINP_LatAccelV_flg/1 -> [VINP_LatAccelV_flg]
  VVMC_LatAccRollAve_Gps/1 -> [VVMC_LatAccRollAve_Gps]
  [VVMC_LatAccRollAve_Gps] -> LateralAccelerationControl/1(VVMC_LatAccRollAve_Gps)
  [VINP_LatAccelV_flg] -> LateralAccelerationControl/2(VINP_LatAccelV_flg)
  LateralAccelerationControl/1(VVMC_LatAccCtrl_flg) -> Cast To Single3/1
  Cast To Single3/1 -> [VVMC_LatAccCtrl_flg]  "VVMC_LatAccCtrl_flg"
  [VVMC_LatAccCtrl_flg] -> SafetyControlJudgement/4(VVMC_LatAccCtrl_flg)
  [VVMC_FrontRearSlipRatioCtrl_flg] -> VVMC_FrontRearSlipRatioCtrl_flg/1
  [VVMC_RearWhlSlipRatioCtrl_flg] -> VVMC_RearWhlSlipRatioCtrl_flg/1
  [VVMC_SingleWhlSlipRatioCtrl_flg] -> VVMC_SingleWhlSlipRatioCtrl_flg/1
  [VVMC_LatAccCtrl_flg] -> VVMC_LatAccCtrl_flg/1
  u2 > 0 (1)/1 -> [VVMC_SafetyCtrl_flg]
  NOT/1 -> Timer/2
  SafetyControlJudgement/1("VVMC_SafetyCtrl_flg ") -> NOT/1, Timer/1
  Constant21/1 -> u2 > 0 (1)/1
  Constant20/1 -> Timer/4, Relational Operator16/2
  Timer/1 -> Relational Operator16/1
  Relational Operator16/1 -> u2 > 0 (1)/2
  Constant22/1 -> u2 > 0 (1)/3
  [task_time_s] -> Timer/3
  VVMC_FeatArbitrFinal_enum/1 -> [VVMC_FeatArbitrFinal_enum]
  [VVMC_FeatArbitrFinal_enum] -> SafetyControlJudgement/5(VVMC_FeatArbitrFinal_enum)
  task_time_s/1 -> [task_time_s]

== system vmc/VMC/VMC/SafetyControl/VehSpdRollingAverage ==
  VVMC_VehicleSpeed_kph : Inport
  task_time_s : Inport  Port=2
  Cast To Single4 : DataTypeConversion  OutDataTypeStr=uint8
  Constant1 : Constant  Value=ZERO_FLOAT
  Constant10 : Constant  Value=ONE_INT
  Constant2 : Constant  Value=KVMC_VehSpdIncSRLim_kphps
  Constant3 : Constant  Value=ONE_INT
  Constant4 : Constant  Value=KVMC_VehSpdRollAveLevel_enum
  Constant5 : Constant  Value=ZERO_FLOAT
  Constant6 : Constant  Value=KVMC_VehSpdDecSRLim_kphps
  Min3 : MinMax  Function=max  Inputs=2
  RateLimit1 : tqr/TQR/Determine Torque Request/TorqueArbitrament/TorqueSmooth/RateLimit
  RollingAverage : Stateflow chart  TreatAsAtomicUnit=on
  VVMC_VehSpdRollAveRaw_kph : Outport
  wires:
  Cast To Single4/1 -> Min3/1
  Min3/1 -> RollingAverage/1(KVMC_VehSpdRollAveLevel_enum)
  Constant10/1 -> Min3/2
  Constant4/1 -> Cast To Single4/1
  Constant5/1 -> RollingAverage/2(ZERO_FLOAT)
  Constant3/1 -> RollingAverage/3(ONE_INT)
  [VVMC_VehicleSpeed_kph] -> RateLimit1/1
  RollingAverage/1(VVMC_VehSpdRollAveRaw_kph) -> [VVMC_VehSpdRollAveRaw_kph]  "VVMC_VehSpdRollAveRaw_kph"
  VVMC_VehicleSpeed_kph/1 -> [VVMC_VehicleSpeed_kph]
  [VVMC_VehSpdRollAveRaw_kph] -> VVMC_VehSpdRollAveRaw_kph/1
  [task_time_s] -> RateLimit1/3
  Constant1/1 -> RateLimit1/2
  Constant2/1 -> RateLimit1/4
  Constant6/1 -> RateLimit1/5
  RateLimit1/1 -> RollingAverage/4(VVMC_VehicleSpeedAftLim_kph)  "VVMC_VehicleSpeedAftLim_kph"
  task_time_s/1 -> [task_time_s]

== system vmc/VMC/VMC/SafetyControl/WheelSpeedRollingAverage ==
  VINP_LFRawWhlSpeed_kph : Inport
  VINP_RFRawWhlSpeed_kph : Inport  Port=2
  VINP_LRRawWhlSpeed_kph : Inport  Port=3
  VINP_RRRawWhlSpeed_kph : Inport  Port=4
  VINP_LFRawWhlSpeedV_flg : Inport  Port=5
  VINP_RFRawWhlSpeedV_flg : Inport  Port=6
  VINP_LRRawWhlSpeedV_flg : Inport  Port=7
  VINP_RRRawWhlSpeedV_flg : Inport  Port=8
  VDDM_ESC1Err_flg : Inport  Port=9
  Cast To Single{1..4} (4 alike) : DataTypeConversion  OutDataTypeStr=uint8
  Constant{1..3,6..7,10,12,16} (8 alike) : Constant  Value=ONE_INT
  Constant{5,9,11,14..15,18..20} (8 alike) : Constant  Value=ZERO_FLOAT
  Constant{4,8,13,17} (4 alike) : Constant  Value=KVMC_WhlSpdRollAveLevel_enum
  Min{,1..3} (4 alike) : MinMax  Function=max  Inputs=2
  OR{,1..3} (4 alike) : Logic  Operator=OR  AllPortsSameDT=off  OutDataTypeStr=boolean
  RollingAverage : Stateflow chart  TreatAsAtomicUnit=on
  RollingAverage1 : Stateflow chart  TreatAsAtomicUnit=on
  RollingAverage2 : Stateflow chart  TreatAsAtomicUnit=on
  RollingAverage3 : Stateflow chart  TreatAsAtomicUnit=on
  Switch{,1..3} (4 alike) : Switch  Criteria=u2 > Threshold
  VVMC_LFWhlSpeedRollAveRaw_kph : Outport
  VVMC_RFWhlSpeedRollAveRaw_kph : Outport  Port=2
  VVMC_LRWhlSpeedRollAveRaw_kph : Outport  Port=3
  VVMC_RRWhlSpeedRollAveRaw_kph : Outport  Port=4
  wires:
  [VINP_RRRawWhlSpeed_kph] -> Switch3/3
  [VINP_RRRawWhlSpeedV_flg] -> OR3/1
  Constant20/1 -> Switch3/1
  [VDDM_ESC1Err_flg] -> OR3/2
  OR3/1 -> Switch3/2
  [VINP_LRRawWhlSpeed_kph] -> Switch2/3
  [VINP_LRRawWhlSpeedV_flg] -> OR2/1
  Constant19/1 -> Switch2/1
  [VDDM_ESC1Err_flg] -> OR2/2
  OR2/1 -> Switch2/2
  [VINP_RFRawWhlSpeed_kph] -> Switch1/3
  [VINP_RFRawWhlSpeedV_flg] -> OR1/1
  Constant15/1 -> Switch1/1
  [VDDM_ESC1Err_flg] -> OR1/2
  OR1/1 -> Switch1/2
  OR/1 -> Switch/2
  [VDDM_ESC1Err_flg] -> OR/2
  VDDM_ESC1Err_flg/1 -> [VDDM_ESC1Err_flg]
  Constant11/1 -> Switch/1
  [VINP_LFRawWhlSpeed_kph] -> Switch/3
  [VINP_LFRawWhlSpeedV_flg] -> OR/1
  VINP_LFRawWhlSpeedV_flg/1 -> [VINP_LFRawWhlSpeedV_flg]
  VINP_RRRawWhlSpeedV_flg/1 -> [VINP_RRRawWhlSpeedV_flg]
  VINP_RFRawWhlSpeedV_flg/1 -> [VINP_RFRawWhlSpeedV_flg]
  VINP_LRRawWhlSpeedV_flg/1 -> [VINP_LRRawWhlSpeedV_flg]
  Cast To Single4/1 -> Min3/1
  Cast To Single3/1 -> Min2/1
  Cast To Single2/1 -> Min1/1
  Cast To Single1/1 -> Min/1
  Constant17/1 -> Cast To Single4/1
  Constant10/1 -> Min3/2
  Constant13/1 -> Cast To Single3/1
  Constant6/1 -> Min2/2
  Constant8/1 -> Cast To Single2/1
  Constant2/1 -> Min1/2
  Constant4/1 -> Cast To Single1/1
  Constant1/1 -> Min/2
  RollingAverage3/1(VVMC_RRWhlSpeedRollAveRaw_kph) -> [VVMC_RRWhlSpeedRollAveRaw_kph]  "VVMC_RRWhlSpeedRollAveRaw_kph"
  RollingAverage1/1(VVMC_RFWhlSpeedRollAveRaw_kph) -> [VVMC_RFWhlSpeedRollAveRaw_kph]  "VVMC_RFWhlSpeedRollAveRaw_kph"
  Min2/1 -> RollingAverage2/1(KVMC_WhlSpdRollAveLevel_enum)
  Constant14/1 -> RollingAverage2/2(ZERO_FLOAT)
  Constant12/1 -> RollingAverage2/3(ONE_INT)
  Switch2/1 -> RollingAverage2/4(VINP_LRRawWhlSpeed_kph)
  RollingAverage2/1(VVMC_LRWhlSpeedRollAveRaw_kph) -> [VVMC_LRWhlSpeedRollAveRaw_kph]  "VVMC_LRWhlSpeedRollAveRaw_kph"
  Switch3/1 -> RollingAverage3/4(VINP_RRRawWhlSpeed_kph)
  Constant16/1 -> RollingAverage3/3(ONE_INT)
  Constant18/1 -> RollingAverage3/2(ZERO_FLOAT)
  Min3/1 -> RollingAverage3/1(KVMC_WhlSpdRollAveLevel_enum)
  Min1/1 -> RollingAverage1/1(KVMC_WhlSpdRollAveLevel_enum)
  Constant9/1 -> RollingAverage1/2(ZERO_FLOAT)
  Constant7/1 -> RollingAverage1/3(ONE_INT)
  Switch1/1 -> RollingAverage1/4(VINP_RFRawWhlSpeed_kph)
  RollingAverage/1(VVMC_LFWhlSpeedRollAveRaw_kph) -> [VVMC_LFWhlSpeedRollAveRaw_kph]  "VVMC_LFWhlSpeedRollAveRaw_kph"
  Switch/1 -> RollingAverage/4(VINP_LFRawWhlSpeed_kph)
  Constant3/1 -> RollingAverage/3(ONE_INT)
  Constant5/1 -> RollingAverage/2(ZERO_FLOAT)
  Min/1 -> RollingAverage/1(KVMC_WhlSpdRollAveLevel_enum)
  VINP_LRRawWhlSpeed_kph/1 -> [VINP_LRRawWhlSpeed_kph]
  VINP_RRRawWhlSpeed_kph/1 -> [VINP_RRRawWhlSpeed_kph]
  VINP_LFRawWhlSpeed_kph/1 -> [VINP_LFRawWhlSpeed_kph]
  VINP_RFRawWhlSpeed_kph/1 -> [VINP_RFRawWhlSpeed_kph]
  [VVMC_LFWhlSpeedRollAveRaw_kph] -> VVMC_LFWhlSpeedRollAveRaw_kph/1
  [VVMC_RFWhlSpeedRollAveRaw_kph] -> VVMC_RFWhlSpeedRollAveRaw_kph/1
  [VVMC_LRWhlSpeedRollAveRaw_kph] -> VVMC_LRWhlSpeedRollAveRaw_kph/1
  [VVMC_RRWhlSpeedRollAveRaw_kph] -> VVMC_RRWhlSpeedRollAveRaw_kph/1

== system vmc/VMC/VMC/Slide Rate  Calculation/4Wheel Calculation ==
  VINP_LFRawWhlSpeed_kph : Inport
  VINP_RFRawWhlSpeed_kph : Inport  Port=2
  VINP_LRRawWhlSpeed_kph : Inport  Port=3
  VINP_RRRawWhlSpeed_kph : Inport  Port=4
  VVMC_LongAcc_Gps : Inport  Port=5
  task_time_s : Inport  Port=6
  VVMC_VehicleSpeed_kph : Inport  Port=7
  VTQD_AfterAvailableTqDemFr_Nm : Inport  Port=8
  VTQD_AfterAvailableTqDemRr_Nm : Inport  Port=9
  VTQD_GearActualPosn_enum : Inport  Port=10
  VINP_LongAccel_Gps : Inport  Port=11
  Constant3 : Constant  Value=KVMC_4WheelLongAccSW_flg
  Determination : Subsystem
  LF Wheel : Subsystem
  LR Wheel : Subsystem
  RF Wheel : Subsystem
  RR Wheel : Subsystem
  Switch : Switch  Criteria=u2 > Threshold
  VVMC_LF4WhlSpdSlideRate_pct : Outport
  VVMC_RF4WhlSpdSlideRate_pct : Outport  Port=2
  VVMC_LR4WhlSpdSlideRate_pct : Outport  Port=3
  VVMC_RR4WhlSpdSlideRate_pct : Outport  Port=4
  VVMC_PredictVehSpd_kph : Outport  Port=5
  VVMC_4WhlSpdSlideRate_pct : Outport  Port=6
  VVMC_AllWhlSkid_flg : Outport  Port=7
  wires:
  [VINP_LongAccel_Gps] -> Switch/1
  [VVMC_LongAcc_Gps] -> Switch/3
  VVMC_LongAcc_Gps/1 -> [VVMC_LongAcc_Gps]
  VINP_LongAccel_Gps/1 -> [VINP_LongAccel_Gps]
  Switch/1 -> [VVMC_4WheelLongAcc_Gps]  "VVMC_4WheelLongAcc_Gps"
  Constant3/1 -> Switch/2
  [VTQD_GearActualPosn_enum] -> LF Wheel/4(VTQD_GearActualPosn_enum)
  [task_time_s] -> LF Wheel/2(task_time_s)
  LF Wheel/3(VVMC_LF4WhlSpdSlideRate_pct) -> [VVMC_LF4WhlSpdSlideRate_pct]
  RF Wheel/3(VVMC_RF4WhlSpdSlideRate_pct) -> [VVMC_RF4WhlSpdSlideRate_pct]
  [VVMC_4WheelLongAcc_Gps] -> LR Wheel/1(VVMC_4WheelLongAcc_Gps)
  [VTQD_GearActualPosn_enum] -> RR Wheel/4(VTQD_GearActualPosn_enum)
  [VVMC_4WheelLongAcc_Gps] -> RR Wheel/1(VVMC_4WheelLongAcc_Gps)
  [VVMC_4WheelLongAcc_Gps] -> Determination/1(VVMC_4WheelLongAcc_Gps)
  RF Wheel/2(VVMC_RFWhlSkid_flg) -> [VVMC_RFWhlSkid_flg]
  LF Wheel/2(VVMC_LFWhlSkid_flg) -> [VVMC_LFWhlSkid_flg]
  [VTQD_AfterAvailableTqDemRr_Nm] -> Determination/14(VTQD_AfterAvailableTqDemRr_Nm)
  [VVMC_RF4WhlSpdSlideRate_pct] -> Determination/10(VVMC_RF4WhlSpdSlideRate_pct)
  [VVMC_LFPreVehSpd_kph] -> Determination/15(VVMC_LFPreVehSpd_kph)
  RR Wheel/2(VVMC_RRWhlSkid_flg) -> [VVMC_RRWhlSkid_flg]
  [VVMC_4WheelLongAcc_Gps] -> RF Wheel/1(VVMC_4WheelLongAcc_Gps)
  LR Wheel/1(VVMC_LRPreVehSpd_kph) -> [VVMC_LRPreVehSpd_kph]
  [VVMC_RFPreVehSpd_kph] -> Determination/16(VVMC_RFPreVehSpd_kph)
  [task_time_s] -> LR Wheel/2(task_time_s)
  RF Wheel/1(VVMC_RFPreVehSpd_kph) -> [VVMC_RFPreVehSpd_kph]
  [VVMC_LRWhlSkid_flg] -> Determination/7(VVMC_LRWhlSkid_flg)
  LR Wheel/2(VVMC_LRWhlSkid_flg) -> [VVMC_LRWhlSkid_flg]
  LR Wheel/3(VVMC_LR4WhlSpdSlideRate_pct) -> [VVMC_LR4WhlSpdSlideRate_pct]
  [VVMC_RFWhlSkid_flg] -> Determination/6(VVMC_RFWhlSkid_flg)
  Determination/3(VVMC_4WhlSpdSlideRate_pct) -> [VVMC_4WhlSpdSlideRate_pct]
  Determination/1(VVMC_PredictVehSpd_kph) -> [VVMC_PredictVehSpd_kph]
  Determination/2(VVMC_AllWhlSkid_flg) -> [VVMC_AllWhlSkid_flg]
  [VVMC_RRPreVehSpd_kph] -> Determination/18(VVMC_RRPreVehSpd_kph)
  [VVMC_VehicleSpeed_kph] -> Determination/3(VVMC_VehicleSpeed_kph)
  [VVMC_LFWhlSkid_flg] -> Determination/5(VVMC_LFWhlSkid_flg)
  [task_time_s] -> Determination/2(task_time_s)
  [VTQD_GearActualPosn_enum] -> Determination/4(VTQD_GearActualPosn_enum)
  [VVMC_LR4WhlSpdSlideRate_pct] -> Determination/11(VVMC_LR4WhlSpdSlideRate_pct)
  [VTQD_AfterAvailableTqDemFr_Nm] -> Determination/13(VTQD_AfterAvailableTqDemFr_Nm)
  RR Wheel/3(VVMC_RR4WhlSpdSlideRate_pct) -> [VVMC_RR4WhlSpdSlideRate_pct]
  [VVMC_RR4WhlSpdSlideRate_pct] -> Determination/12(VVMC_RR4WhlSpdSlideRate_pct)
  [task_time_s] -> RF Wheel/2(task_time_s)
  [task_time_s] -> RR Wheel/2(task_time_s)
  [VINP_LFRawWhlSpeed_kph] -> LF Wheel/3(VINP_LFRawWhlSpeed_kph)
  [VVMC_RRWhlSkid_flg] -> Determination/8(VVMC_RRWhlSkid_flg)
  [VVMC_LF4WhlSpdSlideRate_pct] -> Determination/9(VVMC_LF4WhlSpdSlideRate_pct)
  [VTQD_GearActualPosn_enum] -> LR Wheel/4(VTQD_GearActualPosn_enum)
  RR Wheel/1(VVMC_RRPreVehSpd_kph) -> [VVMC_RRPreVehSpd_kph]
  LF Wheel/1(VVMC_LFPreVehSpd_kph) -> [VVMC_LFPreVehSpd_kph]
  [VTQD_GearActualPosn_enum] -> RF Wheel/4(VTQD_GearActualPosn_enum)
  [VINP_RFRawWhlSpeed_kph] -> RF Wheel/3(VINP_RFRawWhlSpeed_kph)
  [VINP_LRRawWhlSpeed_kph] -> LR Wheel/3(VINP_LRRawWhlSpeed_kph)
  [VINP_RRRawWhlSpeed_kph] -> RR Wheel/3(VINP_RRRawWhlSpeed_kph)
  [VVMC_4WheelLongAcc_Gps] -> LF Wheel/1(VVMC_4WheelLongAcc_Gps)
  [VVMC_LRPreVehSpd_kph] -> Determination/17(VVMC_LRPreVehSpd_kph)
  VTQD_GearActualPosn_enum/1 -> [VTQD_GearActualPosn_enum]
  VTQD_AfterAvailableTqDemRr_Nm/1 -> [VTQD_AfterAvailableTqDemRr_Nm]
  VTQD_AfterAvailableTqDemFr_Nm/1 -> [VTQD_AfterAvailableTqDemFr_Nm]
  [VVMC_AllWhlSkid_flg] -> VVMC_AllWhlSkid_flg/1
  VINP_RRRawWhlSpeed_kph/1 -> [VINP_RRRawWhlSpeed_kph]
  VINP_RFRawWhlSpeed_kph/1 -> [VINP_RFRawWhlSpeed_kph]
  VINP_LFRawWhlSpeed_kph/1 -> [VINP_LFRawWhlSpeed_kph]
  VINP_LRRawWhlSpeed_kph/1 -> [VINP_LRRawWhlSpeed_kph]
  [VVMC_LF4WhlSpdSlideRate_pct] -> VVMC_LF4WhlSpdSlideRate_pct/1
  [VVMC_RF4WhlSpdSlideRate_pct] -> VVMC_RF4WhlSpdSlideRate_pct/1
  [VVMC_RR4WhlSpdSlideRate_pct] -> VVMC_RR4WhlSpdSlideRate_pct/1
  [VVMC_LR4WhlSpdSlideRate_pct] -> VVMC_LR4WhlSpdSlideRate_pct/1
  task_time_s/1 -> [task_time_s]
  VVMC_VehicleSpeed_kph/1 -> [VVMC_VehicleSpeed_kph]
  [VVMC_PredictVehSpd_kph] -> VVMC_PredictVehSpd_kph/1
  [VVMC_4WhlSpdSlideRate_pct] -> VVMC_4WhlSpdSlideRate_pct/1

== system vmc/VMC/VMC/Slide Rate  Calculation/Alternative Wheel Slide Calculation ==
  VINP_LFRawWhlSpeed_kph : Inport
  VINP_RFRawWhlSpeed_kph : Inport  Port=2
  VINP_LRRawWhlSpeed_kph : Inport  Port=3
  VINP_RRRawWhlSpeed_kph : Inport  Port=4
  Abs : Abs
  Abs1 : Abs
  Add : Sum  Inputs=+-
  Add1 : Sum  Inputs=+-
  Constant{,3,5,8} (4 alike) : Constant  Value=KVMC_RawWhlSpeedDeadZone_kph
  Constant1 : Constant  Value=ONE_FLOAT
  Constant2 : Constant  Value=ONE_PERCENT
  Constant4 : Constant  Value=ZERO_FLOAT
  Constant6 : Constant  Value=ONE_FLOAT
  Constant7 : Constant  Value=ONE_PERCENT
  Constant9 : Constant  Value=ZERO_FLOAT
  Divide : Product  Inputs=*//
  Divide1 : Product  Inputs=*//
  Relational Operator{,1..3} (4 alike) : RelationalOperator  Operator=<=  OutDataTypeStr=boolean  RndMeth=Simplest
  Relational Operator4 : RelationalOperator  OutDataTypeStr=boolean  RndMeth=Simplest
  Switch{,1..4} (5 alike) : Switch  Criteria=u2 > Threshold
  VVMC_AltLWhlSlideRate_pct : Outport
  VVMC_AltRWhlSlideRate_pct : Outport  Port=2
  VVMC_AltWhlSlideRate_pct : Outport  Port=3
  wires:
  [VVMC_AltRWhlSlideRate_pct] -> VVMC_AltRWhlSlideRate_pct/1
  Relational Operator2/1 -> Switch2/2
  Switch2/1 -> Divide1/3
  Divide1/1 -> Switch3/3  "VVMC_CalAltRWhlSlideRate_pct"
  Constant5/1 -> Relational Operator2/2
  Constant8/1 -> Relational Operator3/2
  [VINP_RFRawWhlSpeed_kph] -> Relational Operator2/1
  [VINP_LRRawWhlSpeed_kph] -> Add/1
  [VINP_LFRawWhlSpeed_kph] -> Relational Operator/1
  Add1/1 -> Divide1/1
  [VINP_RFRawWhlSpeed_kph] -> Switch2/3
  [VINP_RFRawWhlSpeed_kph] -> Relational Operator3/1
  [VINP_RRRawWhlSpeed_kph] -> Add1/1
  Abs1/1 -> Relational Operator4/2
  [VINP_LFRawWhlSpeed_kph] -> Relational Operator1/1
  Constant/1 -> Relational Operator/2
  Add/1 -> Divide/1
  [VINP_RFRawWhlSpeed_kph] -> Add1/2
  [VVMC_AltWhlSlideRate_pct] -> VVMC_AltWhlSlideRate_pct/1
  Relational Operator/1 -> Switch/2
  [VINP_LFRawWhlSpeed_kph] -> Switch/3
  Constant9/1 -> Switch3/1
  Switch/1 -> Divide/3
  Constant7/1 -> Divide1/2
  Constant2/1 -> Divide/2
  Switch4/1 -> [VVMC_AltWhlSlideRate_pct]  "VVMC_AltWhlSlideRate_pct"
  [VVMC_AltLWhlSlideRate_pct] -> Switch4/1
  [VVMC_AltRWhlSlideRate_pct] -> Abs1/1
  Constant3/1 -> Relational Operator1/2
  Constant4/1 -> Switch1/1
  Switch3/1 -> [VVMC_AltRWhlSlideRate_pct]  "VVMC_AltRWhlSlideRate_pct"
  [VVMC_AltRWhlSlideRate_pct] -> Switch4/3
  VINP_RFRawWhlSpeed_kph/1 -> [VINP_RFRawWhlSpeed_kph]
  VINP_LRRawWhlSpeed_kph/1 -> [VINP_LRRawWhlSpeed_kph]
  VINP_LFRawWhlSpeed_kph/1 -> [VINP_LFRawWhlSpeed_kph]
  [VVMC_AltLWhlSlideRate_pct] -> VVMC_AltLWhlSlideRate_pct/1
  [VVMC_AltLWhlSlideRate_pct] -> Abs/1
  Relational Operator4/1 -> Switch4/2
  Relational Operator3/1 -> Switch3/2
  Constant6/1 -> Switch2/1
  Switch1/1 -> [VVMC_AltLWhlSlideRate_pct]  "VVMC_AltLWhlSlideRate_pct"
  [VINP_LFRawWhlSpeed_kph] -> Add/2
  Constant1/1 -> Switch/1
  Divide/1 -> Switch1/3  "VVMC_CalAltLWhlSlideRate_pct"
  Abs/1 -> Relational Operator4/1
  Relational Operator1/1 -> Switch1/2
  VINP_RRRawWhlSpeed_kph/1 -> [VINP_RRRawWhlSpeed_kph]
